simulink subsystem "Main"  (R2025b)
settings: Solver=VariableStepAuto  StartTime=0.0  StopTime=10.0  RelTol=1e-3
undefined symbols (not defined in the file): Aero_balance, Aeromaps_ON, air_density, Balance_R_11, Br_coef_of_friction_F, Br_coef_of_friction_R, Br_pistons_area_F, Br_pistons_area_R, CdA, CdA_R_11, ClA, ClA_R_11, CoG_z, Default_Fz_FL, Default_Fz_FR, Default_Fz_RL, Default_Fz_RR, Effective_br_disk_r_F, Effective_br_disk_r_R, Front_brake_balance, Front_brake_pump_area, Front_desired_brake_p_balance, Fx, Fy, Fz, g, Gear_ratio, Iz_wehicle, Iz_wheel, Lf, LLTD, Lock_brake_balance, Lr, Mass, Motor_maximum_power, PRT_efficiency, Rear_brake_pump_area, Roll_Angle_11, SA, SR, start_acc_x, start_acc_y, start_velocity_x, start_velocity_y, start_yaw_acc, start_yaw_rate, Static_Camber_FL, Static_Camber_FR, Static_Camber_RL, Static_Camber_RR, Static_Toe_FL, Static_Toe_FR, Static_Toe_RL, Static_Toe_RR, Steering_Angle_FL, Steering_Angle_FR, Steering_Wheel_Angle, Tire_pressure_FL, Tire_pressure_FR, Tire_pressure_RL ... (+18)
libraries: simulink_extras x9, simulink x7
(part 1 of 3)
settings Model: Creator=rafwar4858  LastModifiedBy=rafwar4858

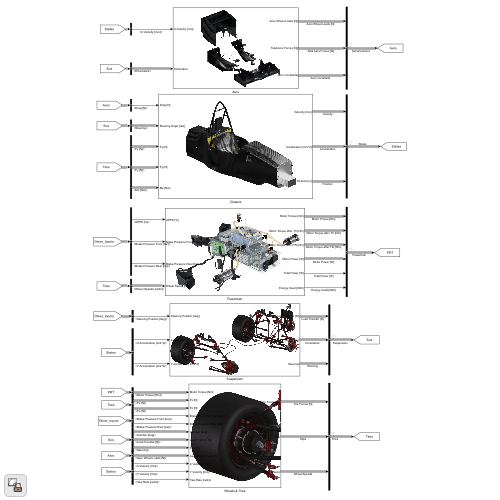
[thumbnail: Simulink's stored preview of the top-level diagram]
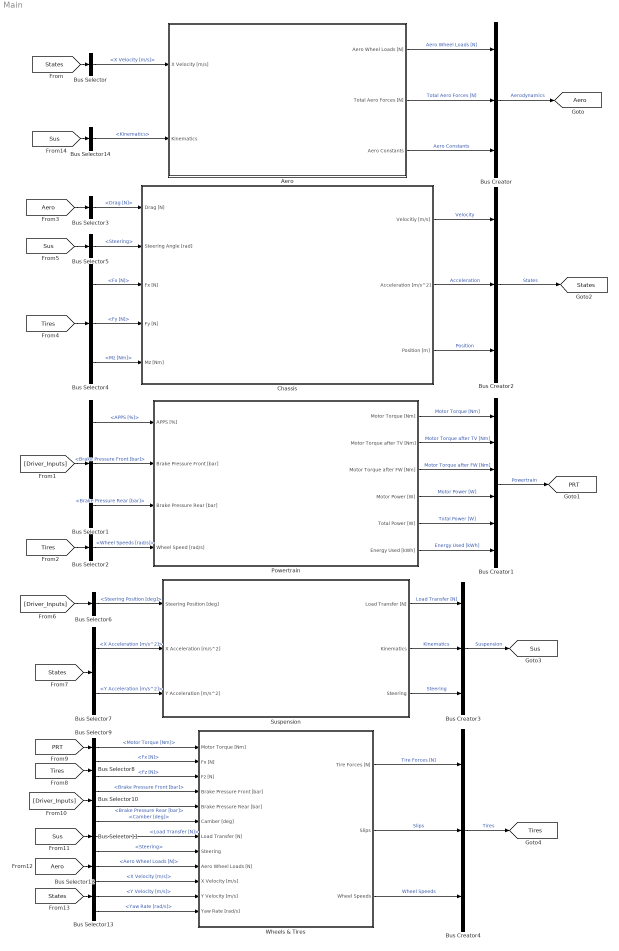
== system Main ==
  Aero : Subsystem
      mask Display: image('aero_rt15.png');
  Bus Creator{,2..4} (4 alike) : BusCreator  Inputs=3
  Bus Creator1 : BusCreator  Inputs=6
  Bus Selector : BusSelector  OutputSignals=Velocity.X Velocity [m/s]
  Bus Selector1 : BusSelector  OutputSignals=APPS [%],Brake Pressure [bar].Brake Pressure Front [bar],Brake Pressure [bar].Brake Pressure Rear [bar]
  Bus Selector10 : BusSelector  OutputSignals=Brake Pressure [bar].Brake Pressure Front [bar],Brake Pressure [bar].Brake Pressure Rear [bar]
  Bus Selector11 : BusSelector  OutputSignals=Kinematics.Camber [deg],Load Transfer [N],Steering
  Bus Selector12 : BusSelector  OutputSignals=Aero Wheel Loads [N]
  Bus Selector13 : BusSelector  OutputSignals=Velocity.X Velocity [m/s],Velocity.Y Velocity [m/s],Velocity.Yaw Rate [rad/s]
  Bus Selector14 : BusSelector  OutputSignals=Kinematics
  Bus Selector2 : BusSelector  OutputSignals=Wheel Speeds.Wheel Speeds [rad/s]
  Bus Selector3 : BusSelector  OutputSignals=Total Aero Forces [N].Drag [N]
  Bus Selector4 : BusSelector  OutputSignals=Tire Forces [N].Fx [N],Tire Forces [N].Fy [N],Tire Forces [N].Mz [Nm]
  Bus Selector5 : BusSelector  OutputSignals=Steering
  Bus Selector6 : BusSelector  OutputSignals=Steering Position [deg]
  Bus Selector7 : BusSelector  OutputSignals=Acceleration.X Acceleration [m/s^2],Acceleration.Y Acceleration [m/s^2]
  Bus Selector8 : BusSelector  OutputSignals=Tire Forces [N].Fx [N],Tire Forces [N].Fz [N]
  Bus Selector9 : BusSelector  OutputSignals=Motor Torque [Nm]
  Chassis : Subsystem
      mask Display: image('monocoque.png');
  Powertrain : Subsystem
      mask Display: image('PRT.png');
  Suspension : Subsystem
      mask Display: image('sus.png');
  Wheels & Tires : Subsystem
      mask Display: image('wheel_rt15e.png');
  tag scope: Aero=global, PRT=global, States=global, Sus=global, Tires=global
  wires:
  Bus Selector4/2 -> Chassis/4(Fy [N])  "<Fy [N]>"
  [States] -> Bus Selector7/1
  Wheels & Tires/2(Slips) -> Bus Creator4/2  "Slips"
  [Sus] -> Bus Selector5/1
  Bus Selector3/1 -> Chassis/1(Drag [N])  "<Drag [N]>"
  Bus Selector8/1 -> Wheels & Tires/2(Fx [N])  "<Fx [N]>"
  Aero/3(Aero Constants) -> Bus Creator/3  "Aero Constants"
  Suspension/2(Kinematics) -> Bus Creator3/2  "Kinematics"
  Powertrain/6(Energy Used [kWh]) -> Bus Creator1/6  "Energy Used [kWh]"
  Bus Creator3/1 -> [Sus]  "Suspension"
  Powertrain/2(Motor Torque after TV [Nm]) -> Bus Creator1/2  "Motor Torque after TV [Nm]"
  Bus Selector/1 -> Aero/1(X Velocity [m/s])  "<X Velocity [m/s]>"
  Bus Creator1/1 -> [PRT]  "Powertrain"
  Bus Selector7/2 -> Suspension/3(Y Acceleration [m/s^2])  "<Y Acceleration [m/s^2]>"
  Bus Selector11/1 -> Wheels & Tires/6(Camber [deg])  "<Camber [deg]>"
  Chassis/1(Velocitiy [m/s]) -> Bus Creator2/1  "Velocity"
  Wheels & Tires/1(Tire Forces [N[) -> Bus Creator4/1  "Tire Forces [N]"
  [States] -> Bus Selector13/1
  Bus Selector7/1 -> Suspension/2(X Acceleration [m/s^2])  "<X Acceleration [m/s^2]>"
  Powertrain/3(Motor Torque after FW [Nm]) -> Bus Creator1/3  "Motor Torque after FW [Nm]"
  [Tires] -> Bus Selector8/1
  Suspension/3(Steering) -> Bus Creator3/3  "Steering"
  Chassis/2(Acceleration [m/s^2]) -> Bus Creator2/2  "Acceleration"
  Aero/2(Total Aero Forces [N]) -> Bus Creator/2  "Total Aero Forces [N]"
  Wheels & Tires/3(Wheel Speeds) -> Bus Creator4/3  "Wheel Speeds"
  Chassis/3(Position [m]) -> Bus Creator2/3  "Position"
  Powertrain/5(Total Power [W]) -> Bus Creator1/5  "Total Power [W]"
  Bus Creator/1 -> [Aero]  "Aerodynamics"
  Suspension/1(Load Transfer [N]) -> Bus Creator3/1  "Load Transfer [N]"
  Bus Selector13/1 -> Wheels & Tires/10(X Velocity [m/s])  "<X Velocity [m/s]>"
  [Aero] -> Bus Selector12/1
  Bus Selector5/1 -> Chassis/2(Steering Angle [rad])  "<Steering>"
  Bus Selector12/1 -> Wheels & Tires/9(Aero Wheel Loads [N])  "<Aero Wheel Loads [N]>"
  Powertrain/1(Motor Torque [Nm]) -> Bus Creator1/1  "Motor Torque [Nm]"
  Bus Selector14/1 -> Aero/2(Kinematics)  "<Kinematics>"
  Powertrain/4(Motor Power [W]) -> Bus Creator1/4  "Motor Power [W]"
  [Tires] -> Bus Selector4/1
  Bus Selector2/1 -> Powertrain/4(Wheel Speed [rad/s])  "<Wheel Speeds [rad/s]>"
  [Sus] -> Bus Selector11/1
  Bus Selector11/2 -> Wheels & Tires/7(Load Transfer [N])  "<Load Transfer [N]>"
  Bus Selector4/1 -> Chassis/3(Fx [N])  "<Fx [N]>"
  [PRT] -> Bus Selector9/1
  [Sus] -> Bus Selector14/1
  Bus Selector4/3 -> Chassis/5(Mz [Nm])  "<Mz [Nm]>"
  Bus Selector13/3 -> Wheels & Tires/12(Yaw Rate [rad/s])  "<Yaw Rate [rad/s]>"
  Bus Creator2/1 -> [States]  "States"
  Bus Selector9/1 -> Wheels & Tires/1(Motor Torque [Nm])  "<Motor Torque [Nm]>"
  Bus Selector11/3 -> Wheels & Tires/8(Steering)  "<Steering>"
  Bus Selector8/2 -> Wheels & Tires/3(Fz [N])  "<Fz [N]>"
  Aero/1(Aero Wheel Loads [N]) -> Bus Creator/1  "Aero Wheel Loads [N]"
  Bus Selector13/2 -> Wheels & Tires/11(Y Velocity [m/s])  "<Y Velocity [m/s]>"
  [States] -> Bus Selector/1
  [Tires] -> Bus Selector2/1
  [Aero] -> Bus Selector3/1
  Bus Creator4/1 -> [Tires]  "Tires"
  [Driver_Inputs] -> Bus Selector1/1
  Bus Selector1/1 -> Powertrain/1(APPS [%])  "<APPS [%]>"
  Bus Selector1/2 -> Powertrain/2(Brake Pressure Front [bar])  "<Brake Pressure Front [bar]>"
  Bus Selector1/3 -> Powertrain/3(Brake Pressure Rear [bar])  "<Brake Pressure Rear [bar]>"
  [Driver_Inputs] -> Bus Selector6/1
  Bus Selector6/1 -> Suspension/1(Steering Position [deg])  "<Steering Position [deg]>"
  [Driver_Inputs] -> Bus Selector10/1
  Bus Selector10/1 -> Wheels & Tires/4(Brake Pressure Front [bar])  "<Brake Pressure Front [bar]>"
  Bus Selector10/2 -> Wheels & Tires/5(Brake Pressure Rear [bar])  "<Brake Pressure Rear [bar]>"

== system Main/Aero ==
  X Velocity [m/s] : Inport
  Kinematics : Inport  Port=2
  Constants Calculation : Subsystem
      settings: PortSchema="{\"entries\":[{\"content\":{\"sides\":[{\"content\":{},\"type\":\"ConnectorPlacement.EquallySpacedRectSide\",\"uuid\":\"1d1f6237-3d99-4612-976d-71cb16498aa4\"},{\"content\":{\"connectorIds\":[\"Out1\"],\"side\":\"RIGHT\"},\"type\":\"ConnectorPlacement.EquallySpacedRectSide\",\"uuid\":\"ace4a0a1-2349-4d5d-abce-6f7f9b544118\"},{\"content\":{\"connectorIds\":[\"In1\"],\"side\":\"TOP\"},\"type\":\"ConnectorPlacement.EquallySpacedRectSide\",\"uuid\":\"df1c56c6-da11-4e38-934f-b242b64638fa\"}]},\"type\":\"ConnectorPlacement.EquallySpacedConnector\",\"uuid\":\"4d4282ef-f96b-4a57-8976-50540634d367\"}],\"packageUris\":[\"http://schema.mathworks.com/mf0/Connector/R2020b\"],\"version\":\"1.0\"}"
  Subsystem : Subsystem
  Total Aero Forces Calculation : Subsystem
      settings: PortSchema="{\"entries\":[{\"content\":{\"sides\":[{\"content\":{\"connectorIds\":[\"In1\"]},\"type\":\"ConnectorPlacement.EquallySpacedRectSide\",\"uuid\":\"0e38cab3-b70b-4fcc-93ca-648bb6f7f98d\"},{\"content\":{\"connectorIds\":[\"Out1\"],\"side\":\"RIGHT\"},\"type\":\"ConnectorPlacement.EquallySpacedRectSide\",\"uuid\":\"d6c16347-4c2c-4bec-93a8-590221b003ca\"},{\"content\":{\"connectorIds\":[\"In2\"],\"side\":\"TOP\"},\"type\":\"ConnectorPlacement.EquallySpacedRectSide\",\"uuid\":\"25fc275c-3a3c-4584-9b78-314a034d51e1\"}]},\"type\":\"ConnectorPlacement.EquallySpacedConnector\",\"uuid\":\"3c4e3b0c-9f26-4570-bbb4-cb0e69afd711\"}],\"packageUris\":[\"http://schema.mathworks.com/mf0/Connector/R2020b\"],\"version\":\"1.0\"}"
  Aero Wheel Loads [N] : Outport
  Total Aero Forces [N] : Outport  Port=2
  Aero Constants : Outport  Port=3
  wires:
  Kinematics/1 -> Constants Calculation/1(Kinematics)
  X Velocity [m/s]/1 -> Total Aero Forces Calculation/2(X Velocity [m/s])  "X Velocity [m/s]"
  Subsystem/1(Aero Wheel Loads [N]) -> Aero Wheel Loads [N]/1  "Aero Wheel Loads [N]"
  Total Aero Forces Calculation/1(Total Aero Forces [N]) -> Subsystem/1(Total Aero Forces [N]), Total Aero Forces [N]/1  "Total Aero Forces [N]"
  Constants Calculation/1(Aero Constants) -> Total Aero Forces Calculation/1(Aero Constants), Aero Constants/1  "Aero Constants"

== system Main/Chassis ==
  Drag [N] : Inport
  Steering Angle [rad] : Inport  Port=2
  Fx [N] : Inport  Port=3
  Fy [N] : Inport  Port=4
  Mz [Nm] : Inport  Port=5
  Acceleration Calculation : Subsystem
  Bus Creator1 : BusCreator  Inputs=3
  Bus Creator2 : BusCreator  Inputs=3
  Bus Creator4 : BusCreator  Inputs=3
  Position Calculation : Subsystem
  Velocitiy Calculation : Subsystem
  Velocitiy [m/s] : Outport
  Acceleration [m/s^2] : Outport  Port=2
  Position [m] : Outport  Port=3
  wires:
  Mz [Nm]/1 -> Acceleration Calculation/5(Mz [Nm])
  Fy [N]/1 -> Acceleration Calculation/4(Fy [N])
  Fx [N]/1 -> Acceleration Calculation/3(Fx [N])
  Steering Angle [rad]/1 -> Acceleration Calculation/2(Steering Angle [rad])
  Drag [N]/1 -> Acceleration Calculation/1(Drag [N])
  Position Calculation/3(Yaw angle [rad]) -> Bus Creator4/3
  Bus Creator4/1 -> Position [m]/1  "Position [m]"
  Position Calculation/2(Y Position [m]) -> Bus Creator4/2
  Position Calculation/1(X Position [m]) -> Bus Creator4/1
  Acceleration Calculation/2(Y Acceleration [m/s^2]) -> Bus Creator1/2, Velocitiy Calculation/2(Y Acceleration [m/s^2])
  Acceleration Calculation/1(X Acceleration [m/s^2]) -> Velocitiy Calculation/1(X Acceleration [m/s^2]), Bus Creator1/1
  Velocitiy Calculation/3(Yaw Rate [rad/s]) -> Bus Creator2/3
  Velocitiy Calculation/2(Y Velocity [m/s]) -> Bus Creator2/2
  Velocitiy Calculation/1(X Velocity [m/s]) -> Bus Creator2/1
  Acceleration Calculation/3(Yaw Acceleration [rad/s^2]) -> Bus Creator1/3, Velocitiy Calculation/3(Yaw Acceleration [rad/s^2])
  Bus Creator1/1 -> Acceleration [m/s^2]/1  "Acceleration [m/s^2]"
  Bus Creator2/1 -> Velocitiy [m/s]/1  "Velocitiy [m/s]"

== system Main/Powertrain ==
  APPS [%] : Inport
  Brake Pressure Front [bar] : Inport  Port=2
  Brake Pressure Rear [bar] : Inport  Port=3
  Wheel Speed [rad/s] : Inport  Port=4
  Energy Calculation : Subsystem
  Motors : Subsystem
  Motor Torque [Nm] : Outport
  Motor Torque after TV [Nm] : Outport  Port=2
  Motor Torque after FW [Nm] : Outport  Port=3
  Motor Power [W] : Outport  Port=4
  Total Power [W] : Outport  Port=5
  Energy Used [kWh] : Outport  Port=6
  wires:
  Brake Pressure Rear [bar]/1 -> Motors/3(Brake Pressure Rear [bar])
  Motors/3(Motor Torque after FW [Nm]) -> Motor Torque after FW [Nm]/1  "Motor Torque after FW [Nm]"
  Motors/2(Motor Torque after TV [Nm]) -> Motor Torque after TV [Nm]/1  "Motor Torque after TV [Nm]"
  APPS [%]/1 -> Motors/1(APPS [%])
  Brake Pressure Front [bar]/1 -> Motors/2(Brake Pressure Front [bar])
  Wheel Speed [rad/s]/1 -> Motors/4(Wheel Speed [rad/s])
  Energy Calculation/1(Total Power [W]) -> Total Power [W]/1  "Total Power [W]"
  Energy Calculation/2(Energy Used [kWh]) -> Energy Used [kWh]/1  "Energy Used [kWh]"
  Motors/1(Motor Torque [Nm]) -> Motor Torque [Nm]/1  "Motor Torque [Nm]"
  Motors/4(Motor Power [W]) -> Energy Calculation/1(Motor Power [W]), Motor Power [W]/1  "Motor Power [W]"

== system Main/Suspension ==
  Steering Position [deg] : Inport
  X Acceleration [m/s^2] : Inport  Port=2
  Y Acceleration [m/s^2] : Inport  Port=3
  "Kinematics " : Subsystem
  Load Transfer : Subsystem
  "Steering " : Subsystem
  Load Transfer [N] : Outport
  Kinematics : Outport  Port=2
  Steering : Outport  Port=3
  wires:
  Y Acceleration [m/s^2]/1 -> Load Transfer/2(Y Acceleration [m/s^2]), "Kinematics "/2(Y Acceleration [m/s^2])
  X Acceleration [m/s^2]/1 -> Load Transfer/1(X Acceleration [m/s^2]), "Kinematics "/1(X Acceleration [m/s^2])
  "Steering "/1(Steering) -> Steering/1  "Steering"
  Load Transfer/1(Load Transfer [N]) -> Load Transfer [N]/1  "Load Transfer [N]"
  "Kinematics "/1(Kinematics) -> "Steering "/1(Kinematics), Kinematics/1  "Kinematics"
  Steering Position [deg]/1 -> "Steering "/2(Steering Position [deg])

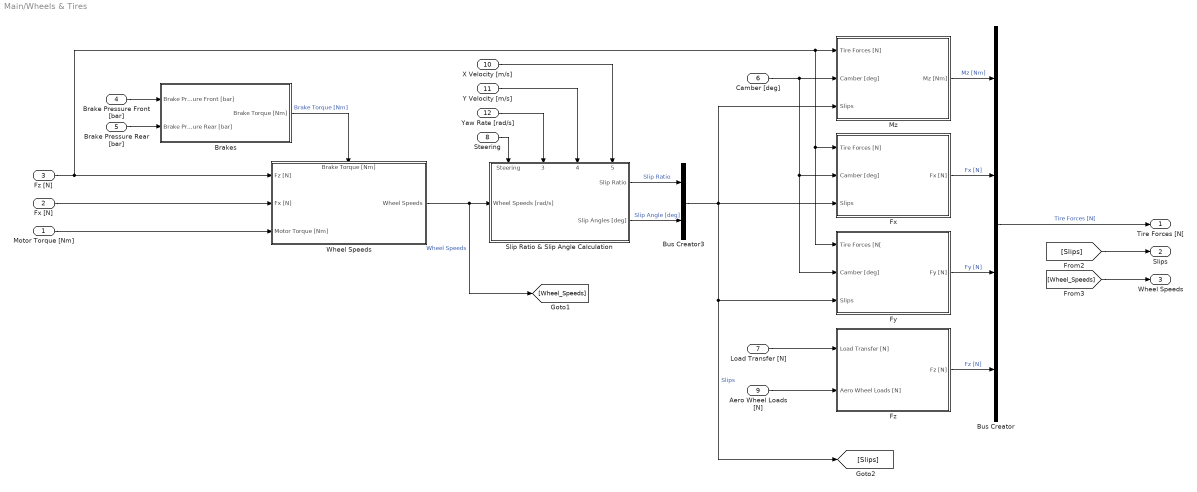
== system Main/Wheels & Tires ==
  Motor Torque [Nm] : Inport
  Fx [N] : Inport  Port=2
  Fz [N] : Inport  Port=3
  Brake Pressure Front [bar] : Inport  Port=4
  Brake Pressure Rear [bar] : Inport  Port=5
  Camber [deg] : Inport  Port=6
  Load Transfer [N] : Inport  Port=7
  Steering : Inport  Port=8
  Aero Wheel Loads [N] : Inport  Port=9
  X Velocity [m/s] : Inport  Port=10
  Y Velocity [m/s] : Inport  Port=11
  Yaw Rate [rad/s] : Inport  Port=12
  Brakes : Subsystem
  Bus Creator : BusCreator  Inputs=4
  Bus Creator3 : BusCreator  Inputs=2
  Fx : Subsystem
  Fy : Subsystem
  Fz : Subsystem
  Mz : Subsystem
  Slip Ratio & Slip Angle Calculation : Subsystem
      settings: PortSchema="{\"entries\":[{\"content\":{\"sides\":[{\"content\":{\"connectorIds\":[\"In1\"]},\"type\":\"ConnectorPlacement.EquallySpacedRectSide\",\"uuid\":\"6298232f-d9bf-440e-9a5a-28adbbbaec2c\"},{\"content\":{\"connectorIds\":[\"Out1\",\"Out2\"],\"side\":\"RIGHT\"},\"type\":\"ConnectorPlacement.EquallySpacedRectSide\",\"uuid\":\"4523207a-72de-4fd2-bf41-45861732d1e3\"},{\"content\":{\"connectorIds\":[\"In2\",\"In3\",\"In4\",\"In5\"],\"side\":\"TOP\"},\"type\":\"ConnectorPlacement.EquallySpacedRectSide\",\"uuid\":\"0cdfbd43-93f5-42d9-8883-a227b445fecf\"}]},\"type\":\"ConnectorPlacement.EquallySpacedConnector\",\"uuid\":\"d3b20827-182e-4fca-a496-83a254f5c692\"}],\"packageUris\":[\"http://schema.mathworks.com/mf0/Connector/R2020b\"],\"version\":\"1.0\"}"
  "Wheel Speeds " : Subsystem
      settings: PortSchema="{\"entries\":[{\"content\":{\"sides\":[{\"content\":{\"connectorIds\":[\"In1\",\"In2\",\"In3\"]},\"type\":\"ConnectorPlacement.EquallySpacedRectSide\",\"uuid\":\"124e436b-f64c-4028-8095-1d8f772c4fa3\"},{\"content\":{\"connectorIds\":[\"Out1\"],\"side\":\"RIGHT\"},\"type\":\"ConnectorPlacement.EquallySpacedRectSide\",\"uuid\":\"9f40d3b5-88bb-42e4-84dd-7d55a8f5d4b6\"},{\"content\":{\"connectorIds\":[\"In4\"],\"side\":\"TOP\"},\"type\":\"ConnectorPlacement.EquallySpacedRectSide\",\"uuid\":\"9d151df8-d681-4246-ac1a-4865a41edfc5\"}]},\"type\":\"ConnectorPlacement.EquallySpacedConnector\",\"uuid\":\"843c1e6a-deb6-4dbc-8d76-71cc70acac89\"}],\"packageUris\":[\"http://schema.mathworks.com/mf0/Connector/R2020b\"],\"version\":\"1.0\"}"
  Tire Forces [N[ : Outport
  Slips : Outport  Port=2
  Wheel Speeds : Outport  Port=3
  wires:
  Steering/1 -> Slip Ratio & Slip Angle Calculation/2(Steering)
  Yaw Rate [rad/s]/1 -> Slip Ratio & Slip Angle Calculation/3(Yaw Rate [rad/s])
  Y Velocity [m/s]/1 -> Slip Ratio & Slip Angle Calculation/4(Y Velocity [m/s])
  X Velocity [m/s]/1 -> Slip Ratio & Slip Angle Calculation/5(X Velocity [m/s])
  Fz [N]/1 -> Mz/1(Tire Forces [N]), Fx/1(Tire Forces [N]), Fy/1(Tire Forces [N[), "Wheel Speeds "/1(Fz [N])
  Camber [deg]/1 -> Fx/2(Camber [deg]), Fy/2(Camber [deg]), Mz/2(Camber [deg])
  Aero Wheel Loads [N]/1 -> Fz/2(Aero Wheel Loads [N])
  Load Transfer [N]/1 -> Fz/1(Load Transfer [N])
  Brake Pressure Rear [bar]/1 -> Brakes/2(Brake Pressure Rear [bar])
  Brake Pressure Front [bar]/1 -> Brakes/1(Brake Pressure Front [bar])
  Fx [N]/1 -> "Wheel Speeds "/2(Fx [N])
  Motor Torque [Nm]/1 -> "Wheel Speeds "/3(Motor Torque [Nm])
  Mz/1(Mz [Nm]) -> Bus Creator/1  "Mz [Nm]"
  [Wheel_Speeds] -> Wheel Speeds/1
  [Slips] -> Slips/1
  Brakes/1(Brake Torque [Nm]) -> "Wheel Speeds "/4(Brake Torque [Nm])  "Brake Torque [Nm]"
  Bus Creator/1 -> Tire Forces [N[/1  "Tire Forces [N["
  "Wheel Speeds "/1(Wheel Speeds) -> Slip Ratio & Slip Angle Calculation/1(Wheel Speeds [rad/s]), [Wheel_Speeds]  "Wheel Speeds"
  Fz/1(Fz [N]) -> Bus Creator/4  "Fz [N]"
  Bus Creator3/1 -> Fx/3(Slips), Mz/3(Slips), Fy/3(Slips), [Slips]  "Slips"
  Fy/1(Fy [N]) -> Bus Creator/3  "Fy [N]"
  Fx/1(Fx [N]) -> Bus Creator/2  "Fx [N]"
  Slip Ratio & Slip Angle Calculation/2(Slip Angles [deg]) -> Bus Creator3/2  "Slip Angle [deg]"
  Slip Ratio & Slip Angle Calculation/1(Slip Ratio) -> Bus Creator3/1  "Slip Ratio"

== system Main/Aero/Constants Calculation ==
  Kinematics : Inport
  Aero Balance : Lookup_n-D  NumberOfTableDimensions=1  BreakpointsForDimension1=Roll_Angle_11  Table=Balance_R_11  InternalRulePriority=Speed  RndMeth=Simplest
  Bus Creator : BusCreator  Inputs=3
  Bus Creator1 : BusCreator  Inputs=3
  Bus Selector : BusSelector  OutputSignals=Pitch,Roll
  Constant : Constant  Value=Aeromaps_ON
  Constant1 : Constant  Value=Aero_balance
  Constant2 : Constant  Value=CdA
  Constant3 : Constant  Value=ClA
  Downforce : Lookup_n-D  NumberOfTableDimensions=1  BreakpointsForDimension1=Roll_Angle_11  Table=ClA_R_11  InternalRulePriority=Speed  RndMeth=Simplest
  Drag : Lookup_n-D  NumberOfTableDimensions=1  BreakpointsForDimension1=Roll_Angle_11  Table=CdA_R_11  InternalRulePriority=Speed  RndMeth=Simplest
  Switch : Switch  Criteria=u2 > Threshold  SaturateOnIntegerOverflow=off  InputSameDT=off
  Aero Constants : Outport
  wires:
  Bus Selector/2 -> Drag/1, Downforce/1, Aero Balance/1  "<Roll>"
  Kinematics/1 -> Bus Selector/1
  Switch/1 -> Aero Constants/1  "Aero Constants"
  Bus Creator/1 -> Switch/1
  Constant1/1 -> Bus Creator1/3  "Aero Balance [%]"
  Constant3/1 -> Bus Creator1/2  "ClA"
  Downforce/1 -> Bus Creator/2  "ClA"
  Constant2/1 -> Bus Creator1/1  "CdA"
  Constant/1 -> Switch/2
  Bus Creator1/1 -> Switch/3
  Aero Balance/1 -> Bus Creator/3  "Aero Balance [%]"
  Drag/1 -> Bus Creator/1  "CdA"

== system Main/Aero/Subsystem ==
  Total Aero Forces [N] : Inport
  Bus Creator : BusCreator  Inputs=4
  Bus Selector : BusSelector  OutputSignals=Downforce Front [N],Downforce Rear [N]
  Gain{1..4} (4 alike) : Gain  Gain=1/2
  Aero Wheel Loads [N] : Outport
  wires:
  Gain1/1 -> Bus Creator/1  "Aero Load FL [N]"
  Gain2/1 -> Bus Creator/3  "Aero Load RL [N]"
  Gain4/1 -> Bus Creator/4  "Aero Load RR [N]"
  Gain3/1 -> Bus Creator/2  "Aero Load FR [N]"
  Total Aero Forces [N]/1 -> Bus Selector/1
  Bus Creator/1 -> Aero Wheel Loads [N]/1  "Aero Wheel Loads [N]"
  Bus Selector/1 -> Gain3/1, Gain1/1  "<Downforce Front [N]>"
  Bus Selector/2 -> Gain2/1, Gain4/1  "<Downforce Rear [N]>"

== system Main/Aero/Total Aero Forces Calculation ==
  Aero Constants : Inport
  X Velocity [m/s] : Inport  Port=2
  Bus Creator2 : BusCreator  Inputs=4
  Bus Selector1 : BusSelector  OutputSignals=CdA,ClA,Aero Balance [%]
  Gain : Gain  Gain=0.01
  Gain1 : Gain  Gain=air_density
  Gain2 : Gain  Gain=1/2
  Product : Product
  Product1 : Product
  Product2 : Product
  Square : Math  Operator=square
  Subtract1 : Sum  Inputs=+-
  Total Aero Forces [N] : Outport
  wires:
  Gain/1 -> Product2/2
  Gain2/1 -> Product/2, Product1/1
  Product1/1 -> Subtract1/1, Bus Creator2/2, Product2/1  "Downforce [N]"
  Bus Selector1/3 -> Gain/1  "<Aero Balance [%]>"
  Square/1 -> Gain1/1
  Subtract1/1 -> Bus Creator2/3  "Downforce Rear [N]"
  Bus Selector1/1 -> Product/1  "<CdA>"
  X Velocity [m/s]/1 -> Square/1  "X Velocity [m/s]"
  Bus Selector1/2 -> Product1/2  "<ClA>"
  Gain1/1 -> Gain2/1
  Product2/1 -> Bus Creator2/4, Subtract1/2  "Downforce Front [N]"
  Product/1 -> Bus Creator2/1  "Drag [N]"
  Bus Creator2/1 -> Total Aero Forces [N]/1  "Total Aero Forces [N]"
  Aero Constants/1 -> Bus Selector1/1

== system Main/Chassis/Acceleration Calculation ==
  note: Fx [N]
  Drag [N] : Inport
  Steering Angle [rad] : Inport  Port=2
  Fx [N] : Inport  Port=3
  Fy [N] : Inport  Port=4
  Mz [Nm] : Inport  Port=5
  IC : InitialCondition  Value=start_yaw_acc
  IC1 : InitialCondition  Value=start_acc_y
  IC2 : InitialCondition  Value=start_acc_x
  Lateral Acceleration : Subsystem
  Longitudinal Acceleration : Subsystem
  Memory : Memory  InheritSampleTime=on
  Memory1 : Memory  InheritSampleTime=on
  Memory2 : Memory  InheritSampleTime=on
  To Workspace1 : ToWorkspace  VariableName=acc_y  SaveFormat=Structure With Time  SampleTime=-1
  To Workspace2 : ToWorkspace  VariableName=acc_x  SaveFormat=Structure With Time  SampleTime=-1
  To Workspace3 : ToWorkspace  VariableName=acc_yaw  SaveFormat=Structure With Time  SampleTime=-1
  Yaw_Acceleration : Subsystem
  X Acceleration [m/s^2] : Outport
  Y Acceleration [m/s^2] : Outport  Port=2
  Yaw Acceleration [rad/s^2] : Outport  Port=3
  wires:
  Mz [Nm]/1 -> Yaw_Acceleration/4(Mz [Nm])
  Memory2/1 -> IC/1
  Memory1/1 -> IC1/1
  Memory/1 -> IC2/1
  Yaw_Acceleration/1(Yaw_Acceleration [rad/s^2]) -> Memory2/1  "Yaw Acceleration [rad/s^2]"
  Lateral Acceleration/1(Y Acceleration [m/s^2]) -> Memory1/1  "Y Acceleration [m/s^2]"
  Longitudinal Acceleration/1(X Acceleration [m/s^2]) -> Memory/1  "X Acceleration [m/s2]"
  IC2/1 -> X Acceleration [m/s^2]/1, To Workspace2/1  "X Acceleration [m/s^2]"
  IC1/1 -> Y Acceleration [m/s^2]/1, To Workspace1/1  "Y Acceleration [m/s^2]"
  IC/1 -> Yaw Acceleration [rad/s^2]/1, To Workspace3/1  "Yaw Acceleration [rad/s^2]"
  Drag [N]/1 -> Longitudinal Acceleration/1(Drag [N])
  Fx [N]/1 -> Longitudinal Acceleration/3(Fx [N]), Yaw_Acceleration/2(Fx [N]), Lateral Acceleration/2(Fx [N])
  Fy [N]/1 -> Longitudinal Acceleration/4(Fy [N]), Lateral Acceleration/3(Fy [N]), Yaw_Acceleration/1(Fy [N])
  Steering Angle [rad]/1 -> Longitudinal Acceleration/2(Steering Angle [rad]), Yaw_Acceleration/3(Steering Angle [rad]), Lateral Acceleration/1(Steering Angle [rad])

== system Main/Chassis/Position Calculation ==
  Add : Sum
  Add1 : Sum
  Bus Selector : BusSelector  OutputSignals=Velocity.Yaw Rate [rad/s],Velocity.X Velocity [m/s],Velocity.Y Velocity [m/s]
  Cos : Trigonometry  Operator=cos
  Gain : Gain  Gain=-1
  Integrator : Integrator
  Integrator5 : Integrator
  Integrator7 : Integrator
  Product{,1,4..5} (4 alike) : Product
  Sin : Trigonometry
  X Position [m] : Outport
  Y Position [m] : Outport  Port=2
  Yaw angle [rad] : Outport  Port=3
  wires:
  Bus Selector/2 -> Product5/1, Product/1  "<X Velocity [m/s]>"
  Bus Selector/1 -> Integrator/1  "<Yaw Rate [rad/s]>"
  [States] -> Bus Selector/1
  Product5/1 -> Add/1
  Product4/1 -> Add/2
  Add1/1 -> Integrator7/1
  Gain/1 -> Product4/1
  Product/1 -> Add1/1
  Bus Selector/3 -> Gain/1, Product1/2  "<Y Velocity [m/s]>"
  Add/1 -> Integrator5/1
  Sin/1 -> Product4/2, Product/2
  Cos/1 -> Product1/1, Product5/2
  Product1/1 -> Add1/2
  Integrator5/1 -> X Position [m]/1  "X Position [m]"
  Integrator/1 -> Cos/1, Sin/1, Yaw angle [rad]/1  "Yaw angle [rad]"
  Integrator7/1 -> Y Position [m]/1  "Y Position [m]"

== system Main/Chassis/Velocitiy Calculation ==
  X Acceleration [m/s^2] : Inport
  Y Acceleration [m/s^2] : Inport  Port=2
  Yaw Acceleration [rad/s^2] : Inport  Port=3
  Add2 : Sum
  Atan2 : Trigonometry  Operator=atan2
  Integrator2 : Integrator  InitialCondition=start_velocity_y
  Integrator3 : Integrator  InitialCondition=start_velocity_x
  Integrator4 : Integrator  InitialCondition=start_yaw_rate
  Product2 : Product
  Product3 : Product
  Radians to Degrees : simulink_extras/Transformations/Radians to Degrees
  Saturation : Saturate  UpperLimit=inf  LowerLimit=0.2
  Subtract1 : Sum  Inputs=-+
  Terminator : Terminator
  Terminator1 : Terminator
  To Workspace : ToWorkspace  VariableName=vel_y  SaveFormat=Structure With Time  SampleTime=-1
  To Workspace1 : ToWorkspace  VariableName=vel_x  SaveFormat=Structure With Time  SampleTime=-1
  To Workspace2 : ToWorkspace  VariableName=vel_yaw  SaveFormat=Structure With Time  SampleTime=-1
  X Velocity [m/s] : Outport
  Y Velocity [m/s] : Outport  Port=2
  Yaw Rate [rad/s] : Outport  Port=3
  wires:
  Atan2/1 -> Terminator/1  "Sideslip Angle [deg]"
  Radians to Degrees/1 -> Terminator1/1  "Yaw Rate [deg/s]"
  Saturation/1 -> X Velocity [m/s]/1, [V_x], To Workspace1/1, Atan2/2  "X Velocity [m/s]"
  [V_y] -> Product2/2
  [V_x] -> Product3/1
  Integrator4/1 -> Product3/2, Product2/1, Yaw Rate [rad/s]/1, To Workspace2/1, Radians to Degrees/1  "Yaw Rate [rad/s]"
  X Acceleration [m/s^2]/1 -> Add2/1
  Product3/1 -> Subtract1/1
  Subtract1/1 -> Integrator2/1
  Integrator3/1 -> Saturation/1
  Add2/1 -> Integrator3/1
  Y Acceleration [m/s^2]/1 -> Subtract1/2
  Product2/1 -> Add2/2
  Integrator2/1 -> Y Velocity [m/s]/1, [V_y], To Workspace/1, Atan2/1  "Y Velocity [m/s]"
  Yaw Acceleration [rad/s^2]/1 -> Integrator4/1

== system Main/Powertrain/Energy Calculation ==
  Motor Power [W] : Inport
  Add : Sum  Inputs=4
  Bus Selector : BusSelector  OutputSignals=Motor Power FL [W],Motor Power FR [W],Motor Power RL [W],Motor Power RR [W]
  Gain1 : Gain  Gain=1/3.6e6
  Integrator : Integrator
  Total Power [W] : Outport
  Energy Used [kWh] : Outport  Port=2
  wires:
  Gain1/1 -> Energy Used [kWh]/1  "Energy Used [kWh]"
  Add/1 -> Integrator/1, Total Power [W]/1  "Total Power [W]"
  Bus Selector/4 -> Add/4  "<Motor Power RR [W]>"
  Bus Selector/3 -> Add/3  "<Motor Power RL [W]>"
  Bus Selector/2 -> Add/2  "<Motor Power FR [W]>"
  Bus Selector/1 -> Add/1  "<Motor Power FL [W]>"
  Motor Power [W]/1 -> Bus Selector/1
  Integrator/1 -> Gain1/1  "Energy [J]"

== system Main/Powertrain/Motors ==
  APPS [%] : Inport
  Brake Pressure Front [bar] : Inport  Port=2
  Brake Pressure Rear [bar] : Inport  Port=3
  Wheel Speed [rad/s] : Inport  Port=4
  Add : Sum
  Control Algorithms : Subsystem
      settings: PortSchema="{\"entries\":[{\"content\":{\"sides\":[{\"content\":{\"connectorIds\":[\"In1\"]},\"type\":\"ConnectorPlacement.EquallySpacedRectSide\",\"uuid\":\"ff79468d-d390-40a0-b232-ab99a3923213\"},{\"content\":{\"connectorIds\":[\"Out1\"],\"side\":\"RIGHT\"},\"type\":\"ConnectorPlacement.EquallySpacedRectSide\",\"uuid\":\"fb8b61d8-96f3-446e-9033-90c3302973a8\"},{\"content\":{\"connectorIds\":[\"In2\",\"In3\"],\"side\":\"TOP\"},\"type\":\"ConnectorPlacement.EquallySpacedRectSide\",\"uuid\":\"43fe1afc-c140-4ab9-95eb-408ded4abd1a\"}]},\"type\":\"ConnectorPlacement.EquallySpacedConnector\",\"uuid\":\"8910aceb-832f-413d-ba51-1e0cfb6ef6d4\"}],\"packageUris\":[\"http://schema.mathworks.com/mf0/Connector/R2020b\"],\"version\":\"1.0\"}"
  Field Weakening : Subsystem
      settings: PortSchema="{\"entries\":[{\"content\":{\"sides\":[{\"content\":{\"connectorIds\":[\"In1\"]},\"type\":\"ConnectorPlacement.EquallySpacedRectSide\",\"uuid\":\"3b3b33d2-9ae6-48d2-a3ac-b2e3893c12cb\"},{\"content\":{\"connectorIds\":[\"Out1\"],\"side\":\"RIGHT\"},\"type\":\"ConnectorPlacement.EquallySpacedRectSide\",\"uuid\":\"4334327f-6778-4d20-95bc-d852004d739b\"},{\"content\":{\"connectorIds\":[\"In2\"],\"side\":\"TOP\"},\"type\":\"ConnectorPlacement.EquallySpacedRectSide\",\"uuid\":\"a4ce2ee0-9b24-47fb-aa94-81c65f3c7fbb\"}]},\"type\":\"ConnectorPlacement.EquallySpacedConnector\",\"uuid\":\"69b43874-ca21-4527-96fe-f2b400e98470\"}],\"packageUris\":[\"http://schema.mathworks.com/mf0/Connector/R2020b\"],\"version\":\"1.0\"}"
  Gain : Gain  Gain=PRT_efficiency
  Power Limit : Subsystem
      settings: PortSchema="{\"entries\":[{\"content\":{\"sides\":[{\"content\":{\"connectorIds\":[\"In1\"]},\"type\":\"ConnectorPlacement.EquallySpacedRectSide\",\"uuid\":\"452dd652-5180-4543-ada6-4c5839127c22\"},{\"content\":{\"connectorIds\":[\"Out1\",\"Out2\"],\"side\":\"RIGHT\"},\"type\":\"ConnectorPlacement.EquallySpacedRectSide\",\"uuid\":\"dd569043-7555-4629-b4bf-b00e9b0fc88f\"},{\"content\":{\"connectorIds\":[\"In2\",\"In3\"],\"side\":\"TOP\"},\"type\":\"ConnectorPlacement.EquallySpacedRectSide\",\"uuid\":\"26cb3e44-4379-4a0b-8699-df6253041f33\"}]},\"type\":\"ConnectorPlacement.EquallySpacedConnector\",\"uuid\":\"45064ad5-d063-45bf-a638-15c05fd0d580\"}],\"packageUris\":[\"http://schema.mathworks.com/mf0/Connector/R2020b\"],\"version\":\"1.0\"}"
  Regen Braking : Subsystem
  Torque Command [Nm] : Subsystem
  Motor Torque [Nm] : Outport
  Motor Torque after TV [Nm] : Outport  Port=2
  Motor Torque after FW [Nm] : Outport  Port=3
  Motor Power [W] : Outport  Port=4
  wires:
  Brake Pressure Rear [bar]/1 -> Regen Braking/2(Brake Pressure Rear [bar])
  Wheel Speed [rad/s]/1 -> Field Weakening/2(Wheel Speed [rad/s]), Control Algorithms/3(Wheel Speed [rad/s]), Power Limit/3(Wheel Speed [rad/s])
  Gain/1 -> Field Weakening/1(Torque Command [Nm])
  Power Limit/1(Motor Power [W]) -> Motor Power [W]/1
  Power Limit/2(Motor Torque [Nm]) -> Motor Torque [Nm]/1
  Add/1 -> Gain/1, Control Algorithms/2(Torque Command [Nm]), Power Limit/2("Torque Command {Nm]")  "Torque Command [Nm]"
  Regen Braking/1(Negative Torque Command [Nm]) -> Add/2
  Torque Command [Nm]/1(Positive Torque Command [Nm]) -> Add/1
  APPS [%]/1 -> Torque Command [Nm]/1(APPS [%])
  Brake Pressure Front [bar]/1 -> Regen Braking/1(Brake Pressure Front [bar])
  Control Algorithms/1(Motor Torque after TV [Nm]) -> Power Limit/1(Motor Torque after TV [Nm]), Motor Torque after TV [Nm]/1
  Field Weakening/1(Motor Torque after FW [Nm]) -> Control Algorithms/1(Motor Torque after FW [Nm]), Motor Torque after FW [Nm]/1

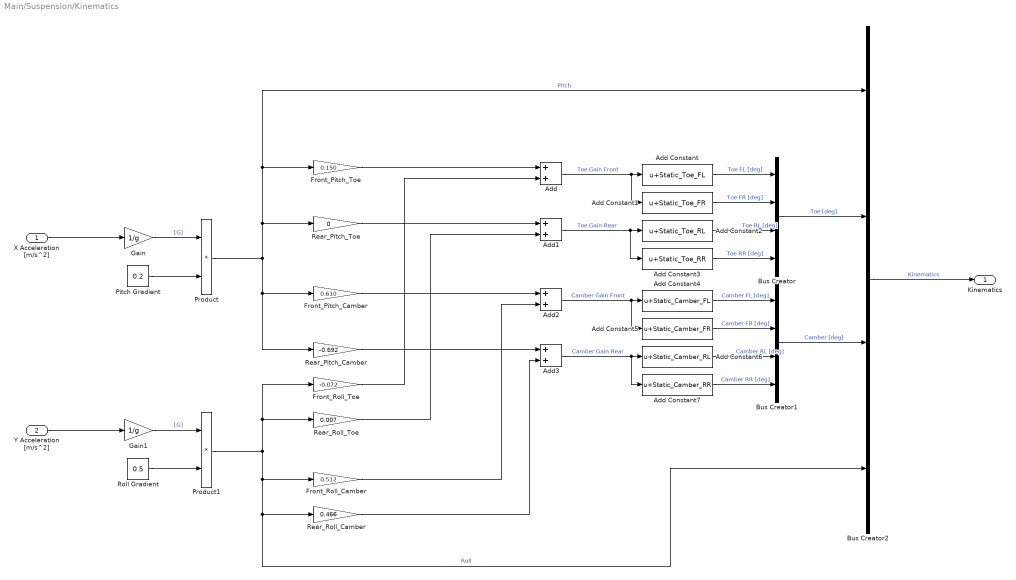
== system Main/Suspension/Kinematics  ==
  X Acceleration [m/s^2] : Inport
  Y Acceleration [m/s^2] : Inport  Port=2
  Add{,1..3} (4 alike) : Sum
  Add Constant : Bias  Bias=Static_Toe_FL  SaturateOnIntegerOverflow=off
  Add Constant1 : Bias  Bias=Static_Toe_FR  SaturateOnIntegerOverflow=off
  Add Constant2 : Bias  Bias=Static_Toe_RL  SaturateOnIntegerOverflow=off
  Add Constant3 : Bias  Bias=Static_Toe_RR  SaturateOnIntegerOverflow=off
  Add Constant4 : Bias  Bias=Static_Camber_FL  SaturateOnIntegerOverflow=off
  Add Constant5 : Bias  Bias=Static_Camber_FR  SaturateOnIntegerOverflow=off
  Add Constant6 : Bias  Bias=Static_Camber_RL  SaturateOnIntegerOverflow=off
  Add Constant7 : Bias  Bias=Static_Camber_RR  SaturateOnIntegerOverflow=off
  Bus Creator : BusCreator  Inputs=4
  Bus Creator1 : BusCreator  Inputs=4
  Bus Creator2 : BusCreator  Inputs=4
  Front_Pitch_Camber : Gain  Gain=0.610
  Front_Pitch_Toe : Gain  Gain=0.150
  Front_Roll_Camber : Gain  Gain=0.512
  Front_Roll_Toe : Gain  Gain=-0.072
  Gain : Gain  Gain=1/g
  Gain1 : Gain  Gain=1/g
  Pitch Gradient : Constant  Value=0.2
  Product : Product
  Product1 : Product
  Rear_Pitch_Camber : Gain  Gain=-0.692
  Rear_Pitch_Toe : Gain  Gain=0
  Rear_Roll_Camber : Gain  Gain=0.466
  Rear_Roll_Toe : Gain  Gain=0.007
  Roll Gradient : Constant  Value=0.5
  Kinematics : Outport
  wires:
  Y Acceleration [m/s^2]/1 -> Gain1/1
  X Acceleration [m/s^2]/1 -> Gain/1
  Add2/1 -> Add Constant4/1, Add Constant5/1  "Camber Gain Front"
  Add3/1 -> Add Constant6/1, Add Constant7/1  "Camber Gain Rear"
  Add Constant4/1 -> Bus Creator1/1  "Camber FL [deg]"
  Add Constant5/1 -> Bus Creator1/2  "Camber FR [deg]"
  Add Constant6/1 -> Bus Creator1/3  "Camber RL [deg]"
  Add Constant7/1 -> Bus Creator1/4  "Camber RR [deg]"
  Bus Creator1/1 -> Bus Creator2/3  "Camber [deg]"
  Bus Creator/1 -> Bus Creator2/2  "Toe [deg]"
  Add Constant3/1 -> Bus Creator/4  "Toe RR [deg]"
  Add Constant2/1 -> Bus Creator/3  "Toe RL [deg]"
  Add Constant1/1 -> Bus Creator/2  "Toe FR [deg]"
  Add Constant/1 -> Bus Creator/1  "Toe FL [deg]"
  Add/1 -> Add Constant/1, Add Constant1/1  "Toe Gain Front"
  Add1/1 -> Add Constant2/1, Add Constant3/1  "Toe Gain Rear"
  Bus Creator2/1 -> Kinematics/1  "Kinematics"
  Roll Gradient/1 -> Product1/2
  Pitch Gradient/1 -> Product/2
  Gain1/1 -> Product1/1  "[G]"
  Front_Pitch_Camber/1 -> Add2/1
  Rear_Roll_Camber/1 -> Add3/2
  Front_Pitch_Toe/1 -> Add/1
  Product/1 -> Rear_Pitch_Camber/1, Front_Pitch_Camber/1, Front_Pitch_Toe/1, Bus Creator2/1, Rear_Pitch_Toe/1  "Pitch"
  Product1/1 -> Rear_Roll_Toe/1, Front_Roll_Toe/1, Front_Roll_Camber/1, Rear_Roll_Camber/1, Bus Creator2/4  "Roll"
  Gain/1 -> Product/1  "[G]"
  Rear_Roll_Toe/1 -> Add1/2
  Front_Roll_Toe/1 -> Add/2
  Rear_Pitch_Toe/1 -> Add1/1
  Front_Roll_Camber/1 -> Add2/2
  Rear_Pitch_Camber/1 -> Add3/1

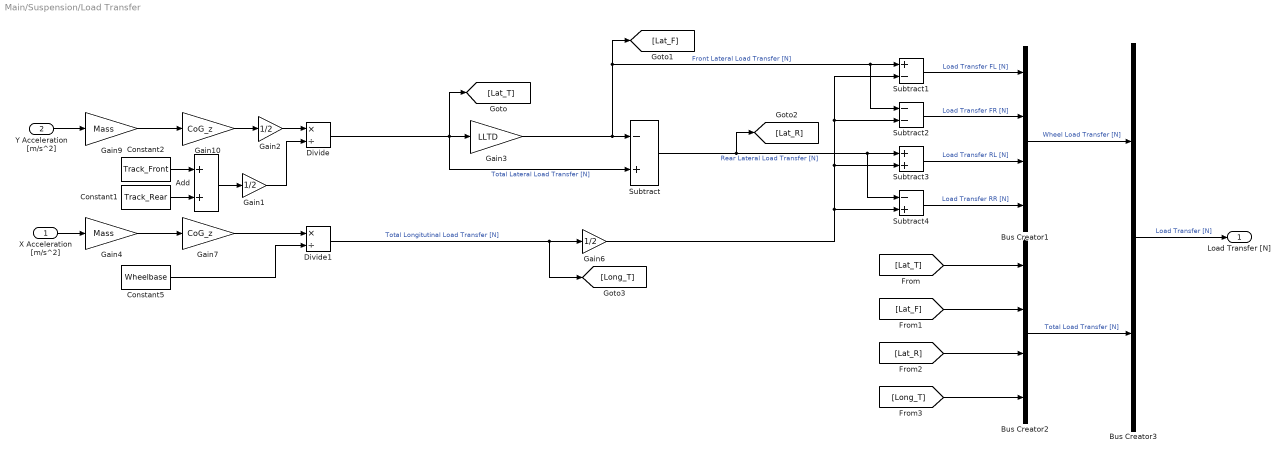
== system Main/Suspension/Load Transfer ==
  X Acceleration [m/s^2] : Inport
  Y Acceleration [m/s^2] : Inport  Port=2
  Add : Sum
  Bus Creator1 : BusCreator  Inputs=4
  Bus Creator2 : BusCreator  Inputs=4
  Bus Creator3 : BusCreator  Inputs=2
  Constant1 : Constant  Value=Track_Rear
  Constant2 : Constant  Value=Track_Front
  Constant5 : Constant  Value=Wheelbase
  Divide : Product  Inputs=*/
  Divide1 : Product  Inputs=*/
  Gain1 : Gain  Gain=1/2
  Gain10 : Gain  Gain=CoG_z
  Gain2 : Gain  Gain=1/2
  Gain3 : Gain  Gain=LLTD
  Gain4 : Gain  Gain=Mass
  Gain6 : Gain  Gain=1/2
  Gain7 : Gain  Gain=CoG_z
  Gain9 : Gain  Gain=Mass
  Subtract : Sum  Inputs=-+
  Subtract1 : Sum  Inputs=+-
  Subtract2 : Sum  Inputs=--
  Subtract3 : Sum
  Subtract4 : Sum  Inputs=-+
  Load Transfer [N] : Outport
  wires:
  X Acceleration [m/s^2]/1 -> Gain4/1
  Y Acceleration [m/s^2]/1 -> Gain9/1
  Gain2/1 -> Divide/1
  Bus Creator3/1 -> Load Transfer [N]/1  "Load Transfer [N]"
  Bus Creator2/1 -> Bus Creator3/2  "Total Load Transfer [N]"
  Bus Creator1/1 -> Bus Creator3/1  "Wheel Load Transfer [N]"
  [Lat_R] -> Bus Creator2/3
  [Lat_T] -> Bus Creator2/1
  [Long_T] -> Bus Creator2/4
  [Lat_F] -> Bus Creator2/2
  Subtract4/1 -> Bus Creator1/4  "Load Transfer RR [N]"
  Subtract3/1 -> Bus Creator1/3  "Load Transfer RL [N]"
  Subtract2/1 -> Bus Creator1/2  "Load Transfer FR [N]"
  Gain6/1 -> Subtract3/2, Subtract2/2, Subtract1/2, Subtract4/2
  Subtract1/1 -> Bus Creator1/1  "Load Transfer FL [N]"
  Subtract/1 -> Subtract3/1, Subtract4/1, [Lat_R]  "Rear Lateral Load Transfer [N]"
  Gain3/1 -> Subtract/1, Subtract2/1, Subtract1/1, [Lat_F]  "Front Lateral Load Transfer [N]"
  Gain10/1 -> Gain2/1
  Add/1 -> Gain1/1
  Constant1/1 -> Add/2
  Gain4/1 -> Gain7/1
  Gain9/1 -> Gain10/1
  Gain7/1 -> Divide1/1
  Divide1/1 -> Gain6/1, [Long_T]  "Total Longitutinal Load Transfer [N]"
  Constant5/1 -> Divide1/2
  Divide/1 -> Gain3/1, Subtract/2, [Lat_T]  "Total Lateral Load Transfer [N]"
  Constant2/1 -> Add/1
  Gain1/1 -> Divide/2

== system Main/Suspension/Steering  ==
  Kinematics : Inport
  Steering Position [deg] : Inport  Port=2
  Add : Sum
  Add1 : Sum
  Bus Creator : BusCreator  Inputs=4
  Bus Creator1 : BusCreator  Inputs=4
  Bus Selector1 : BusSelector  OutputSignals=Toe [deg].Toe FL [deg],Toe [deg].Toe FR [deg],Toe [deg].Toe RL [deg],Toe [deg].Toe RR [deg]
  Degrees to Radians{,1..3} (4 alike) : simulink_extras/Transformations/Degrees to Radians
  FL : Lookup_n-D  NumberOfTableDimensions=1  BreakpointsForDimension1=Steering_Wheel_Angle  Table=Steering_Angle_FL  InternalRulePriority=Speed  RndMeth=Simplest
  FR : Lookup_n-D  NumberOfTableDimensions=1  BreakpointsForDimension1=Steering_Wheel_Angle  Table=Steering_Angle_FR*-1  InternalRulePriority=Speed  RndMeth=Simplest
  Terminator : Terminator
  Steering : Outport
  wires:
  FR/1 -> Add1/1  "Steering Angle FR [deg]"
  FL/1 -> Add/1  "Steering Angle FL [deg]"
  Bus Selector1/4 -> Degrees to Radians3/1, Bus Creator1/4  "<Toe RR [deg]>"
  Bus Selector1/3 -> Degrees to Radians2/1, Bus Creator1/3  "<Toe RL [deg]>"
  Degrees to Radians3/1 -> Bus Creator/4  "Steering Angle RR [rad]"
  Degrees to Radians2/1 -> Bus Creator/3  "Steering Angle RL [rad]"
  Add1/1 -> Degrees to Radians1/1, Bus Creator1/2  "Steering Angle FR [deg]"
  Add/1 -> Bus Creator1/1, Degrees to Radians/1  "Steering Angle FL [deg]"
  Bus Selector1/2 -> Add1/2  "<Toe FR [deg]>"
  Bus Selector1/1 -> Add/2  "<Toe FL [deg]>"
  Kinematics/1 -> Bus Selector1/1
  Bus Creator1/1 -> Terminator/1  "Steering Angle [deg]"
  Degrees to Radians1/1 -> Bus Creator/2  "Steering Angle FR [rad]"
  Degrees to Radians/1 -> Bus Creator/1  "Steering Angle FL [rad]"
  Steering Position [deg]/1 -> FL/1, FR/1  "Steering Position [deg]"
  Bus Creator/1 -> Steering/1  "Steering Angle [rad]"

== system Main/Wheels & Tires/Brakes ==
  Brake Pressure Front [bar] : Inport
  Brake Pressure Rear [bar] : Inport  Port=2
  Brake_Balance_Adjustment : Subsystem
  Braking_Torque_Front : Subsystem
  Braking_Torque_Rear : Subsystem
  Bus Creator2 : BusCreator  Inputs=4
  Gain{,1..3} (4 alike) : Gain  Gain=0.5
  Transfer Fcn : TransferFcn  Denominator=[0.03 1]
  Transfer Fcn1 : TransferFcn  Denominator=[0.03 1]
  Brake Torque [Nm] : Outport
  wires:
  Brake Pressure Rear [bar]/1 -> Transfer Fcn1/1
  Brake Pressure Front [bar]/1 -> Transfer Fcn/1
  Transfer Fcn1/1 -> Braking_Torque_Rear/1(Brake_Pressure [bar])
  Transfer Fcn/1 -> Braking_Torque_Front/1(Brake_Pressure [bar])
  Gain3/1 -> Bus Creator2/4  "Brake Torque RR [Nm]"
  Gain1/1 -> Bus Creator2/2  "Brake Torque FR [Nm]"
  Gain2/1 -> Bus Creator2/3  "Brake Torque RL [Nm]"
  Gain/1 -> Bus Creator2/1  "Brake Torque FL [Nm]"
  Braking_Torque_Rear/1(Braking_Torque [Nm]) -> Brake_Balance_Adjustment/2(Braking_Torque_R [Nm])
  Braking_Torque_Front/1(Braking_torque [Nm]) -> Brake_Balance_Adjustment/1(Braking_Torque_F [Nm])
  Brake_Balance_Adjustment/2(Adj_Braking_Torque_R [Nm]) -> Gain2/1, Gain3/1
  Brake_Balance_Adjustment/1(Adj_Braking_Torque_F [Nm]) -> Gain/1, Gain1/1
  Bus Creator2/1 -> Brake Torque [Nm]/1  "Brake Torque [Nm]"

== system Main/Wheels & Tires/Fx ==
  Tire Forces [N] : Inport
  Camber [deg] : Inport  Port=2
  Slips : Inport  Port=3
  Combined Fx : Subsystem
  Pure Fx NEW : Subsystem  Commented=on
  Pure Fx OLD : Subsystem  Commented=on
  Fx [N] : Outport
  wires:
  Tire Forces [N]/1 -> Combined Fx/1(Tire Forces [N]), Pure Fx NEW/1(Tire Forces [N]), Pure Fx OLD/1(Tire Forces [N])
  Camber [deg]/1 -> Combined Fx/3(Camber [deg]), Pure Fx NEW/3(Camber [deg])
  Combined Fx/1(Fx [N]) -> Fx [N]/1
  Slips/1 -> Combined Fx/2(Slips), Pure Fx NEW/2(Slips), Pure Fx OLD/2(Slips)

== system Main/Wheels & Tires/Fy ==
  Tire Forces [N[ : Inport
  Camber [deg] : Inport  Port=2
  Slips : Inport  Port=3
  Combined Fy : Subsystem
  Pure Fy NEW : Subsystem  Commented=on
  Pure Fy OLD : Subsystem  Commented=on
  Fy [N] : Outport
  wires:
  Slips/1 -> Pure Fy NEW/2(Slips), Pure Fy OLD/2(Slips), Combined Fy/2(Slips)
  Combined Fy/1(Fy [N]) -> Fy [N]/1
  Tire Forces [N[/1 -> Combined Fy/1(Tire Forces [N[), Pure Fy NEW/1(Tire Forces [N[), Pure Fy OLD/1(Tire Forces [N[)
  Camber [deg]/1 -> Combined Fy/3(Camber [deg]), Pure Fy NEW/3(Camber [deg])

== system Main/Wheels & Tires/Fz ==
  Load Transfer [N] : Inport
  Aero Wheel Loads [N] : Inport  Port=2
  Add{,1..3} (4 alike) : Sum  Inputs=+++
  Bus Creator : BusCreator  Inputs=4
  Bus Selector : BusSelector  OutputSignals=Aero Load FL [N]
  Bus Selector1 : BusSelector  OutputSignals=Wheel Load Transfer [N].Load Transfer FL [N]
  Bus Selector2 : BusSelector  OutputSignals=Aero Load FR [N]
  Bus Selector3 : BusSelector  OutputSignals=Wheel Load Transfer [N].Load Transfer FR [N]
  Bus Selector4 : BusSelector  OutputSignals=Aero Load RL [N]
  Bus Selector5 : BusSelector  OutputSignals=Wheel Load Transfer [N].Load Transfer RL [N]
  Bus Selector6 : BusSelector  OutputSignals=Aero Load RR [N]
  Bus Selector7 : BusSelector  OutputSignals=Wheel Load Transfer [N].Load Transfer RR [N]
  Constant1 : Constant  Value=Default_Fz_FR
  Constant2 : Constant  Value=Default_Fz_RL
  Constant3 : Constant  Value=Default_Fz_RR
  Constant5 : Constant  Value=Default_Fz_FL
  Fz [N] : Outport
  wires:
  Bus Selector5/1 -> Add2/2  "<Load Transfer RL [N]>"
  Bus Selector4/1 -> Add2/1  "<Aero Load RL [N]>"
  Bus Selector7/1 -> Add3/2  "<Load Transfer RR [N]>"
  Bus Selector6/1 -> Add3/1  "<Aero Load RR [N]>"
  Aero Wheel Loads [N]/1 -> Bus Selector/1, Bus Selector2/1, Bus Selector4/1, Bus Selector6/1
  Bus Selector2/1 -> Add1/1  "<Aero Load FR [N]>"
  Bus Selector3/1 -> Add1/2  "<Load Transfer FR [N]>"
  Bus Selector1/1 -> Add/2  "<Load Transfer FL [N]>"
  Bus Selector/1 -> Add/1  "<Aero Load FL [N]>"
  Load Transfer [N]/1 -> Bus Selector1/1, Bus Selector3/1, Bus Selector5/1, Bus Selector7/1
  Constant3/1 -> Add3/3
  Constant2/1 -> Add2/3
  Constant1/1 -> Add1/3
  Constant5/1 -> Add/3
  Bus Creator/1 -> Fz [N]/1  "Fz [N]"
  Add/1 -> Bus Creator/1  "Fz FL [N]"
  Add1/1 -> Bus Creator/2  "Fz FR [N]"
  Add2/1 -> Bus Creator/3  "Fz RL [N]"
  Add3/1 -> Bus Creator/4  "Fz RR [N]"

== system Main/Wheels & Tires/Mz ==
  Tire Forces [N] : Inport
  Camber [deg] : Inport  Port=2
  Slips : Inport  Port=3
  Pure Mz : Subsystem
  Mz [Nm] : Outport
  wires:
  Pure Mz/1(Mz [Nm]) -> Mz [Nm]/1
  Slips/1 -> Pure Mz/2(Slips)
  Tire Forces [N]/1 -> Pure Mz/1(Tire Forces [N])
  Camber [deg]/1 -> Pure Mz/3(Camber [deg])

== system Main/Wheels & Tires/Slip Ratio & Slip Angle Calculation ==
  Wheel Speeds [rad/s] : Inport
  Steering : Inport  Port=2
  Yaw Rate [rad/s] : Inport  Port=3
  Y Velocity [m/s] : Inport  Port=4
  X Velocity [m/s] : Inport  Port=5
  Bus Creator1 : BusCreator  Inputs=4
  Bus Selector2 : BusSelector  OutputSignals=Slip Angle FL [rad],Slip Angle FR [rad],Slip Angle RL [rad],Slip Angle RR [rad]
  Radians to Degrees{1..4} (4 alike) : simulink_extras/Transformations/Radians to Degrees
  Saturation{2..5} (4 alike) : Saturate  UpperLimit=0.55  LowerLimit=-0.55
  Slip Angle : Subsystem
  "Slip Ratio " : Subsystem
  Slip Ratio : Outport
  Slip Angles [deg] : Outport  Port=2
  wires:
  Steering/1 -> Slip Angle/4(Steering)
  Yaw Rate [rad/s]/1 -> Slip Angle/2(Yaw Rate [rad/s]), "Slip Ratio "/3(Yaw Rate [rad/s])
  Y Velocity [m/s]/1 -> Slip Angle/3(Y Velocity [m/s])
  X Velocity [m/s]/1 -> Slip Angle/1(X Velocity [m/s]), "Slip Ratio "/2(X Velocity [m/s])
  Saturation5/1 -> Radians to Degrees4/1
  Saturation4/1 -> Radians to Degrees3/1
  Saturation2/1 -> Radians to Degrees2/1
  Saturation3/1 -> Radians to Degrees1/1
  Bus Creator1/1 -> Slip Angles [deg]/1  "Slip Angles"
  Radians to Degrees4/1 -> Bus Creator1/4  "Slip Angle RR [deg]"
  Radians to Degrees3/1 -> Bus Creator1/3  "Slip Angle RL [deg]"
  Radians to Degrees1/1 -> Bus Creator1/1  "Slip Angle FL [deg]"
  Radians to Degrees2/1 -> Bus Creator1/2  "Slip Angle FR [deg]"
  Bus Selector2/4 -> Saturation5/1  "<Slip Angle RR [rad]>"
  Bus Selector2/3 -> Saturation4/1  "<Slip Angle RL [rad]>"
  Bus Selector2/2 -> Saturation2/1  "<Slip Angle FR [rad]>"
  Bus Selector2/1 -> Saturation3/1  "<Slip Angle FL [rad]>"
  Slip Angle/1(Slip Angle [rad]) -> Bus Selector2/1  "Slip Angles"
  Wheel Speeds [rad/s]/1 -> "Slip Ratio "/1(Wheel Speeds [rad/s])
  "Slip Ratio "/1(Slip Ratio) -> Slip Ratio/1  "Slip Ratio"

== system Main/Wheels & Tires/Wheel Speeds  ==
  Fz [N] : Inport
  Fx [N] : Inport  Port=2
  Motor Torque [Nm] : Inport  Port=3
  Brake Torque [Nm] : Inport  Port=4
  Bus Creator : BusCreator  Inputs=4
  Bus Creator1 : BusCreator  Inputs=2
  Bus Creator2 : BusCreator  Inputs=2
  Gain : Gain  Gain=60 / 2 * pi
  Rolling Resistance Calculation : Subsystem
  Wheel Speed FL : Subsystem
  Wheel Speed FR : Subsystem
  Wheel Speed RL : Subsystem
  Wheel Speed RR : Subsystem
  Wheel Speeds : Outport
  wires:
  Bus Creator2/1 -> Wheel Speeds/1  "Wheel Speeds"
  Gain/1 -> Bus Creator2/2  "Wheel Speeds [rpm]"
  Bus Creator1/1 -> Wheel Speed FL/3(Torque [Nm]), Wheel Speed FR/3(Torque [Nm]), Wheel Speed RL/3(Torque [Nm]), Wheel Speed RR/3(Torque [Nm])  "Torque [Nm]"
  Rolling Resistance Calculation/1(Rolling Resistance) -> Wheel Speed FL/1(Rolling Resistance), Wheel Speed FR/1(Rolling Resistance), Wheel Speed RL/1(Rolling Resistance), Wheel Speed RR/1(Rolling Resistance)
  Brake Torque [Nm]/1 -> Bus Creator1/1
  Motor Torque [Nm]/1 -> Bus Creator1/2
  Fz [N]/1 -> Rolling Resistance Calculation/1(Fz [N])
  Wheel Speed RR/1(Wheel Speed RL [rad/s]) -> Bus Creator/4  "Wheel Speed RR [rad/s]"
  Wheel Speed RL/1(Wheel Speed RL [rad/s]) -> Bus Creator/3  "Wheel Speed RL [rad/s]"
  Wheel Speed FL/1(Wheel Speed FL [rad/s]) -> Bus Creator/1  "Wheel Speed FL [rad/s]"
  Wheel Speed FR/1(Wheel Speed FR [rad/s]) -> Bus Creator/2  "Wheel Speed FR [rad/s]"
  Bus Creator/1 -> Bus Creator2/1, Gain/1  "Wheel Speeds [rad/s]"
  Fx [N]/1 -> Wheel Speed FL/2(Fx [N]), Wheel Speed FR/2(Fx [N]), Wheel Speed RL/2(Fx [N]), Wheel Speed RR/2(Fx [N])

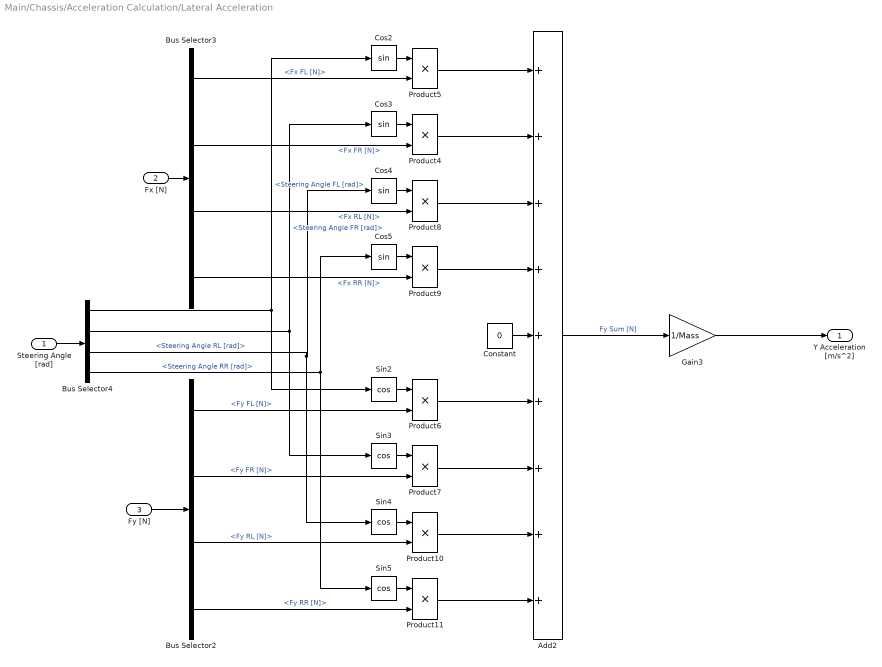
== system Main/Chassis/Acceleration Calculation/Lateral Acceleration ==
  Steering Angle [rad] : Inport
  Fx [N] : Inport  Port=2
  Fy [N] : Inport  Port=3
  Add2 : Sum  Inputs=+++++++++
  Bus Selector2 : BusSelector  OutputSignals=Fy FL [N],Fy FR [N],Fy RL [N],Fy RR [N]
  Bus Selector3 : BusSelector  OutputSignals=Fx FL [N],Fx FR [N],Fx RL [N],Fx RR [N]
  Bus Selector4 : BusSelector  OutputSignals=Steering Angle FL [rad],Steering Angle FR [rad],Steering Angle RL [rad],Steering Angle RR [rad]
  Constant : Constant  Value=0
  Cos{2..5} (4 alike) : Trigonometry
  Gain3 : Gain  Gain=1/Mass
  Product{4..11} (8 alike) : Product
  Sin{2..5} (4 alike) : Trigonometry  Operator=cos
  Y Acceleration [m/s^2] : Outport
  wires:
  Product11/1 -> Add2/9
  Bus Selector2/4 -> Product11/2  "<Fy RR [N]>"
  Product10/1 -> Add2/8
  Bus Selector2/3 -> Product10/2  "<Fy RL [N]>"
  Product9/1 -> Add2/4
  Product8/1 -> Add2/3
  Bus Selector3/4 -> Product9/2  "<Fx RR [N]>"
  Bus Selector3/3 -> Product8/2  "<Fx RL [N]>"
  Constant/1 -> Add2/5
  Bus Selector2/1 -> Product6/2  "<Fy FL [N]>"
  Sin5/1 -> Product11/1
  Bus Selector2/2 -> Product7/2  "<Fy FR [N]>"
  Cos4/1 -> Product8/1
  Bus Selector4/2 -> Cos3/1, Sin3/1  "<Steering Angle FR [rad]>"
  Cos5/1 -> Product9/1
  Bus Selector3/2 -> Product4/2  "<Fx FR [N]>"
  Sin4/1 -> Product10/1
  Sin3/1 -> Product7/1
  Sin2/1 -> Product6/1
  Cos3/1 -> Product4/1
  Product6/1 -> Add2/6
  Product7/1 -> Add2/7
  Product5/1 -> Add2/1
  Cos2/1 -> Product5/1
  Fx [N]/1 -> Bus Selector3/1
  Bus Selector4/1 -> Cos2/1, Sin2/1  "<Steering Angle FL [rad]>"
  Fy [N]/1 -> Bus Selector2/1
  Product4/1 -> Add2/2
  Add2/1 -> Gain3/1  "Fy Sum [N]"
  Gain3/1 -> Y Acceleration [m/s^2]/1
  Bus Selector3/1 -> Product5/2  "<Fx FL [N]>"
  Bus Selector4/4 -> Cos5/1, Sin5/1  "<Steering Angle RR [rad]>"
  Steering Angle [rad]/1 -> Bus Selector4/1
  Bus Selector4/3 -> Cos4/1, Sin4/1  "<Steering Angle RL [rad]>"

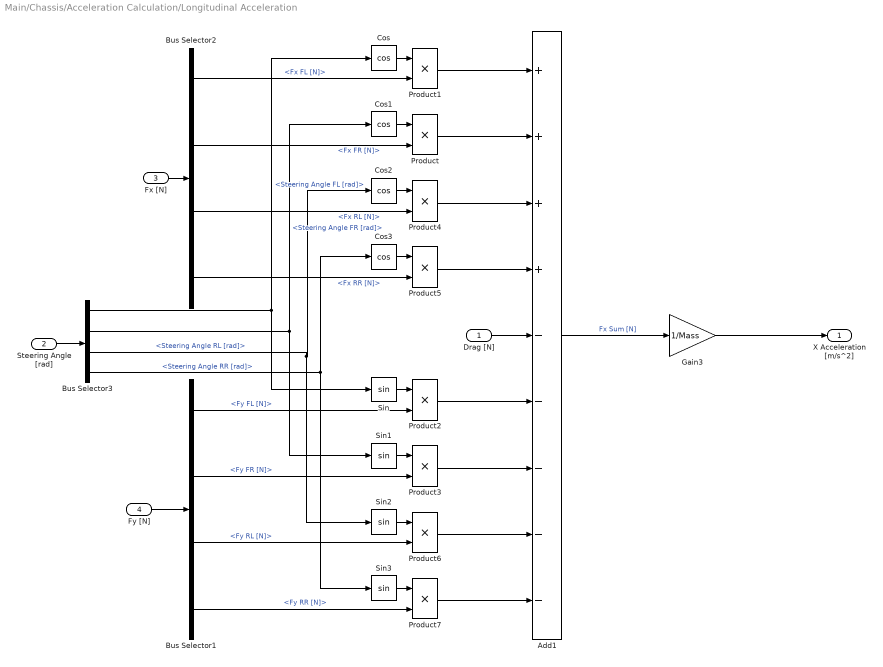
== system Main/Chassis/Acceleration Calculation/Longitudinal Acceleration ==
  Drag [N] : Inport
  Steering Angle [rad] : Inport  Port=2
  Fx [N] : Inport  Port=3
  Fy [N] : Inport  Port=4
  Add1 : Sum  Inputs=++++-----
  Bus Selector1 : BusSelector  OutputSignals=Fy FL [N],Fy FR [N],Fy RL [N],Fy RR [N]
  Bus Selector2 : BusSelector  OutputSignals=Fx FL [N],Fx FR [N],Fx RL [N],Fx RR [N]
  Bus Selector3 : BusSelector  OutputSignals=Steering Angle FL [rad],Steering Angle FR [rad],Steering Angle RL [rad],Steering Angle RR [rad]
  Cos{,1..3} (4 alike) : Trigonometry  Operator=cos
  Gain3 : Gain  Gain=1/Mass
  Product{,1..7} (8 alike) : Product
  Sin{,1..3} (4 alike) : Trigonometry
  X Acceleration [m/s^2] : Outport
  wires:
  Product7/1 -> Add1/9
  Product6/1 -> Add1/8
  Product5/1 -> Add1/4
  Product4/1 -> Add1/3
  Product3/1 -> Add1/7
  Product2/1 -> Add1/6
  Sin2/1 -> Product6/1
  Bus Selector1/3 -> Product6/2  "<Fy RL [N]>"
  Sin3/1 -> Product7/1
  Bus Selector1/4 -> Product7/2  "<Fy RR [N]>"
  Bus Selector1/2 -> Product3/2  "<Fy FR [N]>"
  Sin1/1 -> Product3/1
  Bus Selector1/1 -> Product2/2  "<Fy FL [N]>"
  Sin/1 -> Product2/1
  Drag [N]/1 -> Add1/5
  Cos3/1 -> Product5/1
  Cos2/1 -> Product4/1
  Bus Selector2/4 -> Product5/2  "<Fx RR [N]>"
  Bus Selector2/3 -> Product4/2  "<Fx RL [N]>"
  Bus Selector3/4 -> Cos3/1, Sin3/1  "<Steering Angle RR [rad]>"
  Bus Selector3/3 -> Cos2/1, Sin2/1  "<Steering Angle RL [rad]>"
  Bus Selector3/2 -> Cos1/1, Sin1/1  "<Steering Angle FR [rad]>"
  Bus Selector3/1 -> Cos/1, Sin/1  "<Steering Angle FL [rad]>"
  Gain3/1 -> X Acceleration [m/s^2]/1
  Add1/1 -> Gain3/1  "Fx Sum [N]"
  Bus Selector2/2 -> Product/2  "<Fx FR [N]>"
  Bus Selector2/1 -> Product1/2  "<Fx FL [N]>"
  Fy [N]/1 -> Bus Selector1/1
  Product1/1 -> Add1/1
  Cos/1 -> Product1/1
  Cos1/1 -> Product/1
  Product/1 -> Add1/2
  Fx [N]/1 -> Bus Selector2/1
  Steering Angle [rad]/1 -> Bus Selector3/1
